simulink model "CartesianImpControl"  (R2015b)
settings: Solver=VariableStepAuto  StartTime=0.0  StopTime=10.0  RelTol=1e-3
values from neighbouring files (symbols this model uses):
  dt = dt_sim    (= 0.02)    [ImpControl3Link.m]
  Kd = [50, 50,  0, 0, 0,  50]    [ImpControl3Link.m]
  Kd_env = [200, 200, 0, 0, 0, 0]    [ImpControl3Link.m]
  Kp = [25, 100, 0, 0, 0, 100]    [ImpControl3Link.m]
  Kp_env = [5000, 5000, 0, 0, 0, 0]    [ImpControl3Link.m]
  n = robot.n    [ImpControl3Link.m]
  peg = 1    [ImpControl3Link.m]
  robot = SerialLink([link1, link2, link3], 'name', '3link-robot',     'base',[eye(3), zeros(3,1); zeros(1,3), 1], 'qlim',[-pi, pi; -pi, pi; -pi, pi],     'tool',[eye(3), zeros(3,1); zeros(1,3), 1])    [ImpControl3Link.m]
  xc = [0.45, 2, 2, 10, 10, 10]'    [ImpControl3Link.m]
undefined symbols (not defined in the file or in its folder): jacob_dot, maniplty, mu0
libraries: roblocks x5
settings Model: Creator=victor  LastModifiedBy=victor

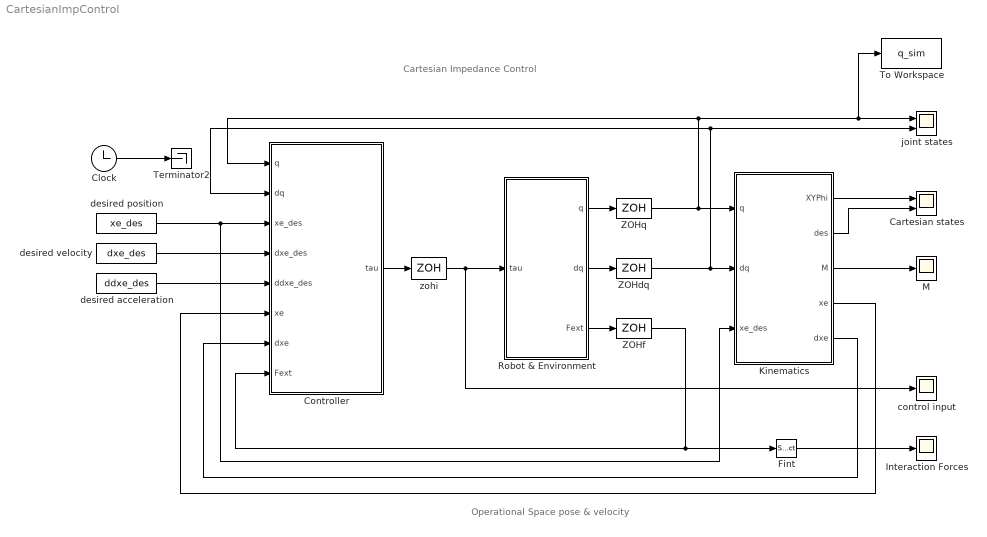
== system CartesianImpControl ==
  note: Operational Space pose & velocity
  note: Cartesian Impedance Control
  Cartesian states : Scope  NumInputPorts=2
  Clock : Clock
  Controller : Subsystem
  Fint : Selector  InputPortWidth=6  IndexOptions=Index vector (dialog)  Indices=[1 2]  OutputSizes=1
  Interaction Forces : Scope
  Kinematics : Subsystem
  M : Scope
  Robot & Environment : Subsystem
  Terminator2 : Terminator
  To Workspace : ToWorkspace  VariableName=q_sim  SampleTime=-1
  ZOHdq : ZeroOrderHold  SampleTime=dt
  ZOHf : ZeroOrderHold  SampleTime=dt
  ZOHq : ZeroOrderHold  SampleTime=dt
  control input : Scope
  desired acceleration : FromWorkspace  VariableName=ddxe_des  SampleTime=dt
  desired position : FromWorkspace  VariableName=xe_des  SampleTime=dt
  desired velocity : FromWorkspace  VariableName=dxe_des  SampleTime=dt
  joint states : Scope  NumInputPorts=2
  zohi : ZeroOrderHold  SampleTime=dt
  wires:
  zohi/1 -> control input/1, Robot & Environment/1(tau)
  Clock/1 -> Terminator2/1
  desired position/1 -> Kinematics/3(xe_des), Controller/3(xe_des)
  Robot & Environment/1(q) -> ZOHq/1
  Robot & Environment/2(dq) -> ZOHdq/1
  ZOHf/1 -> Fint/1, Controller/8(Fext)
  ZOHdq/1 -> Kinematics/2(dq), joint states/2, Controller/2(dq)
  ZOHq/1 -> Kinematics/1(q), To Workspace/1, joint states/1, Controller/1(q)
  desired velocity/1 -> Controller/4(dxe_des)
  desired acceleration/1 -> Controller/5(ddxe_des)
  Controller/1(tau) -> zohi/1
  Kinematics/1(XYPhi) -> Cartesian states/1
  Kinematics/2(des) -> Cartesian states/2
  Kinematics/3(M) -> M/1
  Kinematics/4(xe) -> Controller/6(xe)
  Kinematics/5(dxe) -> Controller/7(dxe)
  Robot & Environment/3(Fext) -> ZOHf/1
  Fint/1 -> Interaction Forces/1

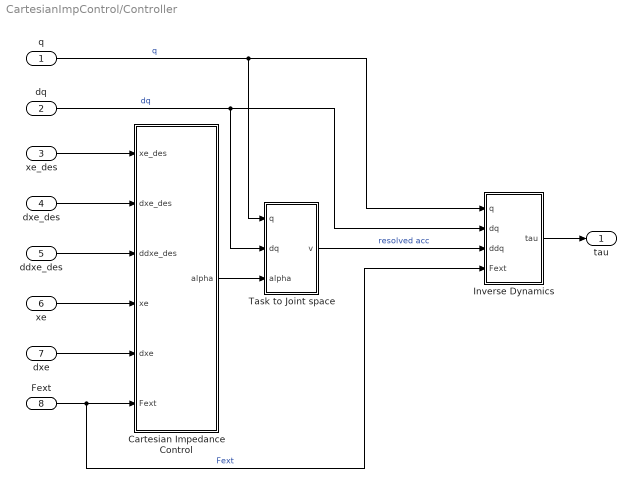
== system CartesianImpControl/Controller ==
  q : Inport
  dq : Inport  Port=2
  xe_des : Inport  Port=3
  dxe_des : Inport  Port=4
  ddxe_des : Inport  Port=5
  xe : Inport  Port=6
  dxe : Inport  Port=7
  Fext : Inport  Port=8
  Cartesian Impedance Control : Subsystem
  Inverse Dynamics : Subsystem
  Task to Joint space : Subsystem
  tau : Outport
  wires:
  dxe_des/1 -> Cartesian Impedance Control/2(dxe_des)
  Cartesian Impedance Control/1(alpha) -> Task to Joint space/3(alpha)
  ddxe_des/1 -> Cartesian Impedance Control/3(ddxe_des)
  Task to Joint space/1(v) -> Inverse Dynamics/3(ddq)  "resolved acc"
  dxe/1 -> Cartesian Impedance Control/5(dxe)
  Inverse Dynamics/1(tau) -> tau/1
  dq/1 -> Task to Joint space/2(dq), Inverse Dynamics/2(dq)  "dq"
  xe/1 -> Cartesian Impedance Control/4(xe)
  Fext/1 -> Inverse Dynamics/4(Fext), Cartesian Impedance Control/6(Fext)  "Fext"
  xe_des/1 -> Cartesian Impedance Control/1(xe_des)
  q/1 -> Inverse Dynamics/1(q), Task to Joint space/1(q)  "q"

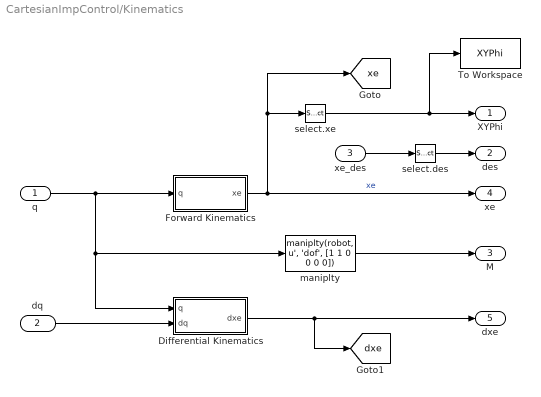
== system CartesianImpControl/Kinematics ==
  q : Inport
  dq : Inport  Port=2
  xe_des : Inport  Port=3
  Differential Kinematics : Subsystem
  Forward Kinematics : Subsystem
  To Workspace : ToWorkspace  VariableName=XYPhi  SaveFormat=Timeseries  SampleTime=-1
  maniplty : MATLABFcn  MATLABFcn=maniplty(robot, u', 'dof', [1 1 0 0 0 0])
  select.des : Selector  InputPortWidth=6  IndexOptions=Index vector (dialog)  Indices=[1 2 6]  OutputSizes=1
  select.xe : Selector  InputPortWidth=6  IndexOptions=Index vector (dialog)  Indices=[1 2 6]  OutputSizes=1
  XYPhi : Outport
  des : Outport  Port=2
  M : Outport  Port=3
  xe : Outport  Port=4
  dxe : Outport  Port=5
  tag scope: dxe=global, xe=global
  wires:
  Forward Kinematics/1(xe) -> xe/1, select.xe/1, [xe]  "xe"
  maniplty/1 -> M/1
  select.des/1 -> des/1
  Differential Kinematics/1(dxe) -> [dxe], dxe/1
  q/1 -> maniplty/1, Differential Kinematics/1(q), Forward Kinematics/1(q)
  dq/1 -> Differential Kinematics/2(dq)
  xe_des/1 -> select.des/1
  select.xe/1 -> To Workspace/1, XYPhi/1

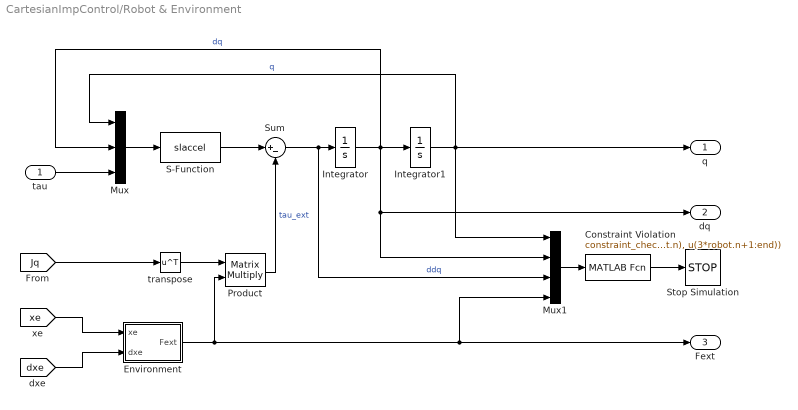
== system CartesianImpControl/Robot & Environment ==
  tau : Inport
  Constraint Violation : MATLABFcn  MATLABFcn=constraint_check(u(1:robot.n), u(robot.n+1:2*robot.n), u(2*robot.n+1:3*robot.n), u(3*robot.n+1:end))
  Environment : Subsystem
  Integrator : Integrator
  Integrator1 : Integrator  InitialCondition=mu0(1:robot.n)
  Mux : Mux  Inputs=3
  Mux1 : Mux
  Product : Product  Multiplication=Matrix(*)
  S-Function : S-Function  FunctionName=slaccel  Parameters=robot  SFunctionDeploymentMode=off  EnableBusSupport=off
  Stop Simulation : Stop
  Sum : Sum  Inputs=|+-
  transpose : Math  Operator=transpose  SaturateOnIntegerOverflow=on
  q : Outport
  dq : Outport  Port=2
  Fext : Outport  Port=3
  wires:
  S-Function/1 -> Sum/1
  Mux/1 -> S-Function/1
  Integrator/1 -> Mux/2, Integrator1/1, Mux1/2, dq/1  "dq"
  tau/1 -> Mux/3
  [Jq] -> transpose/1
  Product/1 -> Sum/2  "tau_ext"
  Integrator1/1 -> Mux1/1, q/1, Mux/1  "q"
  Sum/1 -> Mux1/3, Integrator/1  "ddq"
  transpose/1 -> Product/1
  Mux1/1 -> Constraint Violation/1
  Constraint Violation/1 -> Stop Simulation/1
  [xe] -> Environment/1(xe)
  [dxe] -> Environment/2(dxe)
  Environment/1(Fext) -> Fext/1, Mux1/4, Product/2

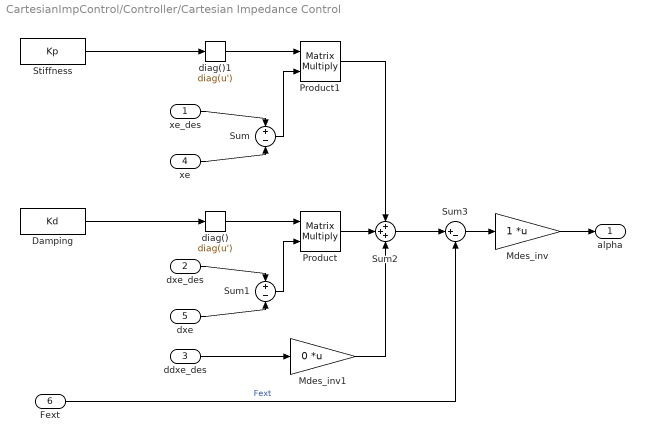
== system CartesianImpControl/Controller/Cartesian Impedance Control ==
  xe_des : Inport
  dxe_des : Inport  Port=2
  ddxe_des : Inport  Port=3
  xe : Inport  Port=4
  dxe : Inport  Port=5
  Fext : Inport  Port=6
  Damping : Constant  Value=Kd
  Mdes_inv : Gain  Multiplication=Matrix(K*u)  SaturateOnIntegerOverflow=on  OutDataTypeStr=Inherit: Same as input  ParamDataTypeStr=Inherit: Same as input
  Mdes_inv1 : Gain  Gain=0  Multiplication=Matrix(K*u)  SaturateOnIntegerOverflow=on  OutDataTypeStr=Inherit: Same as input  ParamDataTypeStr=Inherit: Same as input
  Product : Product  Multiplication=Matrix(*)
  Product1 : Product  Multiplication=Matrix(*)
  Stiffness : Constant  Value=Kp
  Sum : Sum  Inputs=+-  SaturateOnIntegerOverflow=on  InputSameDT=on  OutDataTypeStr=Inherit: Same as first input
  Sum1 : Sum  Inputs=+-  SaturateOnIntegerOverflow=on  InputSameDT=on  OutDataTypeStr=Inherit: Same as first input
  Sum2 : Sum  Inputs=+++  SaturateOnIntegerOverflow=on  InputSameDT=on  OutDataTypeStr=Inherit: Same as first input
  Sum3 : Sum  Inputs=|+-  SaturateOnIntegerOverflow=on  InputSameDT=on  OutDataTypeStr=Inherit: Same as first input
  diag() : MATLABFcn  MATLABFcn=diag(u')  OutputDimensions=[6 6]  Output1D=off
  diag()1 : MATLABFcn  MATLABFcn=diag(u')  OutputDimensions=[6 6]  Output1D=off
  alpha : Outport
  wires:
  xe_des/1 -> Sum/1
  Sum2/1 -> Sum3/1
  Sum3/1 -> Mdes_inv/1
  dxe/1 -> Sum1/2
  xe/1 -> Sum/2
  dxe_des/1 -> Sum1/1
  ddxe_des/1 -> Mdes_inv1/1
  Mdes_inv/1 -> alpha/1
  Damping/1 -> diag()/1
  diag()/1 -> Product/1
  Stiffness/1 -> diag()1/1
  diag()1/1 -> Product1/1
  Sum/1 -> Product1/2
  Product1/1 -> Sum2/1
  Sum1/1 -> Product/2
  Product/1 -> Sum2/2
  Fext/1 -> Sum3/2  "Fext"
  Mdes_inv1/1 -> Sum2/3

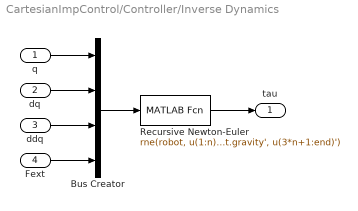
== system CartesianImpControl/Controller/Inverse Dynamics ==
  q : Inport
  dq : Inport  Port=2
  ddq : Inport  Port=3
  Fext : Inport  Port=4
  Bus Creator : BusCreator  Inputs=4
  Recursive Newton-Euler : MATLABFcn  MATLABFcn=rne(robot, u(1:n)', u(n+1:2*n)', u(2*n+1:3*n)', robot.gravity', u(3*n+1:end)')  OutputDimensions=n
  tau : Outport
  wires:
  Recursive Newton-Euler/1 -> tau/1
  q/1 -> Bus Creator/1
  dq/1 -> Bus Creator/2
  ddq/1 -> Bus Creator/3
  Fext/1 -> Bus Creator/4
  Bus Creator/1 -> Recursive Newton-Euler/1

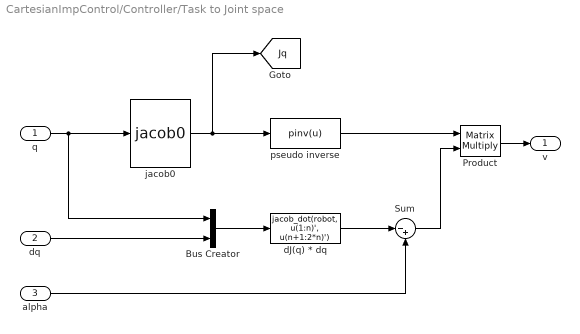
== system CartesianImpControl/Controller/Task to Joint space ==
  q : Inport
  dq : Inport  Port=2
  alpha : Inport  Port=3
  Bus Creator : BusCreator  Inputs=2
  Product : Product  Multiplication=Matrix(*)
  Sum : Sum  Inputs=|-+  SaturateOnIntegerOverflow=on  InputSameDT=on  OutDataTypeStr=Inherit: Same as first input
  dJ(q) * dq : MATLABFcn  MATLABFcn=jacob_dot(robot, u(1:n)', u(n+1:2*n)')  OutputDimensions=[6 1]  Output1D=off
  "jacob0 " : roblocks/Kinematics/jacob0   robot=robot
  pseudo inverse : MATLABFcn  MATLABFcn=pinv(u)  Output1D=off
  v : Outport
  tag scope: Jq=global
  wires:
  "jacob0 "/1 -> [Jq], pseudo inverse/1
  dJ(q) * dq/1 -> Sum/1
  Sum/1 -> Product/2
  Product/1 -> v/1
  pseudo inverse/1 -> Product/1
  q/1 -> Bus Creator/1, "jacob0 "/1
  alpha/1 -> Sum/2
  dq/1 -> Bus Creator/2
  Bus Creator/1 -> dJ(q) * dq/1

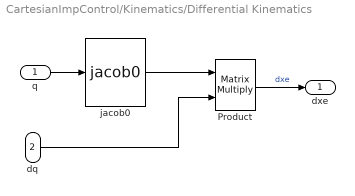
== system CartesianImpControl/Kinematics/Differential Kinematics ==
  q : Inport
  dq : Inport  Port=2
  Product : Product  Multiplication=Matrix(*)
  "jacob0 " : roblocks/Kinematics/jacob0   robot=robot
  dxe : Outport
  wires:
  "jacob0 "/1 -> Product/1
  q/1 -> "jacob0 "/1
  Product/1 -> dxe/1  "dxe"
  dq/1 -> Product/2

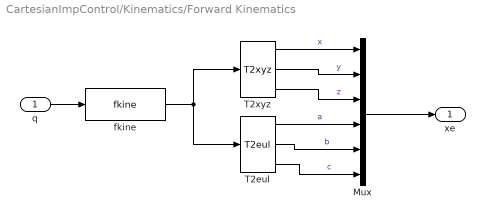
== system CartesianImpControl/Kinematics/Forward Kinematics ==
  q : Inport
  Mux : Mux  Inputs=6
  T2eul : roblocks/Transform Conversion/T2eul
  T2xyz : roblocks/Transform Conversion/T2xyz
  fkine : roblocks/Kinematics/fkine  robot=robot
  xe : Outport
  wires:
  T2xyz/3 -> Mux/3  "z"
  T2eul/3 -> Mux/6  "c"
  T2eul/1 -> Mux/4  "a"
  T2xyz/2 -> Mux/2  "y"
  q/1 -> fkine/1
  fkine/1 -> T2eul/1, T2xyz/1
  T2xyz/1 -> Mux/1  "x"
  T2eul/2 -> Mux/5  "b"
  Mux/1 -> xe/1

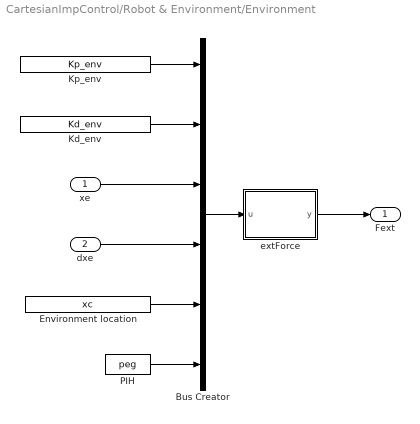
== system CartesianImpControl/Robot & Environment/Environment ==
  xe : Inport
  dxe : Inport  Port=2
  Bus Creator : BusCreator  Inputs=6
  Environment location : Constant  Value=xc  SampleTime=dt
  Kd_env : Constant  Value=Kd_env
  Kp_env : Constant  Value=Kp_env
  PIH : Constant  Value=peg  SampleTime=dt
  extForce : MATLAB Function  TreatAsAtomicUnit=on
  Fext : Outport
  wires:
  Environment location/1 -> Bus Creator/5
  xe/1 -> Bus Creator/3
  Bus Creator/1 -> extForce/1(u)
  Kp_env/1 -> Bus Creator/1
  Kd_env/1 -> Bus Creator/2
  dxe/1 -> Bus Creator/4
  extForce/1(y) -> Fext/1
  PIH/1 -> Bus Creator/6

== matlab function CartesianImpControl/Robot & Environment/Environment/extForce ==
  data: u input; y output
function y = extForcefcn(u)
%#codegen
Fext = zeros(6,1);
Kp_env = u(1:6);
Kd_env = u(7:12);
xe = u(13:18);
dxe = u(19:24);
xc = u(25:30);
peg = u(31);

x_hole = [0.5, 0.3, 0];
r_hole = 0.01;          % tolerance per side of the peg

for i=1:6
    if xe(i) > xc(i)                            % contact
        
        Fext(i) = Kp_env(i)*(xe(i)-xc(i));
        if dxe(i) > 0 
            Fext(i) = Fext(i) + Kd_env(i)*dxe(i);   % damping
        end
    else
        Fext(i) = 0;
    end
end

if peg && xe(2) > x_hole(2)-r_hole && xe(2) < x_hole(2)+r_hole
    Fext(1) = 0;
end

y = Fext;
